simulink model "Batman_symbol"  (R2022a)
settings: Solver=VariableStepAuto  StartTime=0.0  StopTime=8  MaxStep=0.0001  RelTol=1e-3
libraries: simulink x8
settings Model: Creator=Gamer  LastModifiedBy=Gamer
settings SolverCC: ZeroCrossAlgorithm=Adaptive
settings DebuggingCC: IgnoredZcDiagnostic=none

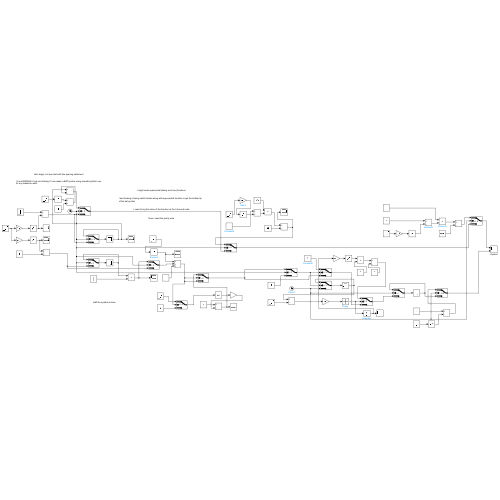
[thumbnail: Simulink's stored preview of the top-level diagram]
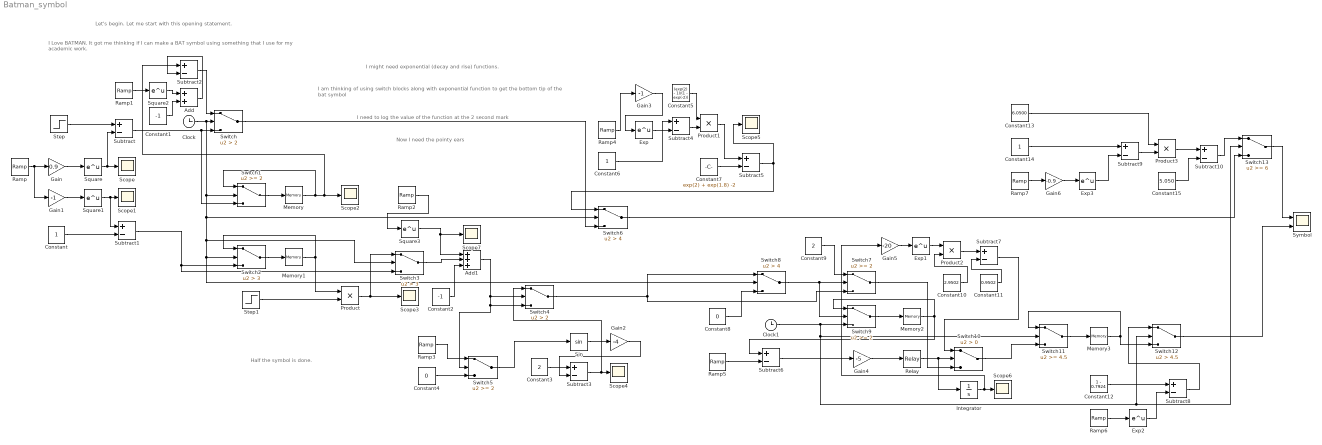
== system Batman_symbol ==
  note: Half the symbol is done.
  note: Now I need the pointy ears
  note: I need to log the value of the function at the 2 second mark
  note: I am thinking of using switch blocks along with exponential function to get the bottom tip of the bat symbol
  note: I might need exponential (decay and rise) functions.
  note: I Love BATMAN. It got me thinking if I can make a BAT symbol using something that I use for my academic work.
  note: Let's begin. Let me start with this opening statement.
  Add : Sum
  Add1 : Sum  Inputs=+++
  Clock : Clock
  Clock1 : Clock
  Constant : Constant
  Constant1 : Constant  Value=-1
  Constant10 : Constant  Value=2.9502
  Constant11 : Constant  Value=0.9502
  Constant12 : Constant  Value=1 - 0.7924
  Constant13 : Constant  Value=6.0500
  Constant14 : Constant
  Constant15 : Constant  Value=5.050
  Constant2 : Constant  Value=-1
  Constant3 : Constant  Value=2
  Constant4 : Constant  Value=0
  Constant5 : Constant  Value=(exp(2) - 1)/(1 - exp(-2))
  Constant6 : Constant
  Constant7 : Constant  Value=exp(2) + exp(1.8) -2
  Constant8 : Constant  Value=0
  Constant9 : Constant  Value=2
  Exp{,1..3} (4 alike) : Math
  Gain : Gain  Gain=0.9
  Gain1 : Gain  Gain=-1
  Gain2 : Gain  Gain=-4
  Gain3 : Gain  Gain=-1
  Gain4 : Gain  Gain=-5
  Gain5 : Gain  Gain=-20
  Gain6 : Gain  Gain=-0.9
  Integrator : Integrator
  Memory{,1..3} (4 alike) : Memory
  Product{,1..3} (4 alike) : Product
  Ramp : simulink/Sources/Ramp  slope=1  start=0  InitialOutput=0
  Ramp1 : simulink/Sources/Ramp  slope=1  start=2  InitialOutput=0
  Ramp2 : simulink/Sources/Ramp  slope=10  start=3.5  InitialOutput=0
  Ramp3 : simulink/Sources/Ramp  slope=4.33  start=0  InitialOutput=0
  Ramp4 : simulink/Sources/Ramp  slope=1  start=4  InitialOutput=0
  Ramp5 : simulink/Sources/Ramp  slope=1  start=0  InitialOutput=0
  Ramp6 : simulink/Sources/Ramp  slope=-0.449  start=4.5  InitialOutput=0
  Ramp7 : simulink/Sources/Ramp  slope=1  start=6  InitialOutput=0
  Relay : Relay  OnSwitchValue=0.001  OffSwitchValue=0
  Scope{,1..7} (8 alike) : Scope
  Sin : Trigonometry
  Square{,1..3} (4 alike) : Math
  Step : Step  Time=0  SampleTime=0
  Step1 : Step  Time=3  SampleTime=0
  Subtract{,1..10} (11 alike) : Sum  Inputs=+-
  Switch : Switch  Criteria=u2 > Threshold  Threshold=2  SaturateOnIntegerOverflow=off  InputSameDT=off
  Switch{1,5,7,9} (4 alike) : Switch  Threshold=2  SaturateOnIntegerOverflow=off  InputSameDT=off
  Switch10 : Switch  Criteria=u2 > Threshold  SaturateOnIntegerOverflow=off  InputSameDT=off
  Switch11 : Switch  Threshold=4.5  SaturateOnIntegerOverflow=off  InputSameDT=off
  Switch12 : Switch  Criteria=u2 > Threshold  Threshold=4.5  SaturateOnIntegerOverflow=off  InputSameDT=off
  Switch13 : Switch  Threshold=6  SaturateOnIntegerOverflow=off  InputSameDT=off
  Switch2 : Switch  Criteria=u2 > Threshold  Threshold=3  SaturateOnIntegerOverflow=off  InputSameDT=off
  Switch3 : Switch  Criteria=u2 > Threshold  Threshold=3  SaturateOnIntegerOverflow=off  InputSameDT=off
  Switch4 : Switch  Criteria=u2 > Threshold  Threshold=2  SaturateOnIntegerOverflow=off  InputSameDT=off
  Switch6 : Switch  Criteria=u2 > Threshold  Threshold=4  SaturateOnIntegerOverflow=off  InputSameDT=off
  Switch8 : Switch  Criteria=u2 > Threshold  Threshold=4  SaturateOnIntegerOverflow=off  InputSameDT=off
  Symbol : Scope  NumInputPorts=2
  wires:
  Step/1 -> Subtract/1
  Ramp/1 -> Gain1/1, Gain/1
  Square/1 -> Scope/1, Subtract/2
  Subtract/1 -> Switch1/3, Switch/3
  Gain/1 -> Square/1
  Gain1/1 -> Square1/1
  Square1/1 -> Subtract1/1, Scope1/1
  Constant/1 -> Subtract1/2
  Subtract1/1 -> Switch3/3, Switch2/3
  Clock/1 -> Switch8/2, Switch2/2, Switch3/2, Switch6/2, Switch1/2, Switch/2
  Ramp1/1 -> Square2/1
  Square2/1 -> Add/1
  Subtract2/1 -> Switch/1
  Switch1/1 -> Memory/1
  Memory/1 -> Subtract2/1, Scope2/1, Switch1/1
  Constant1/1 -> Add/2
  Add/1 -> Subtract2/2
  Switch2/1 -> Memory1/1
  Memory1/1 -> Switch2/1, Product/1
  Step1/1 -> Product/2
  Product/1 -> Switch3/1, Scope3/1
  Switch3/1 -> Add1/2
  Ramp2/1 -> Square3/1
  Square3/1 -> Scope7/1, Add1/1
  Add1/1 -> Switch5/2, Switch4/3, Switch4/2
  Constant2/1 -> Add1/3
  Switch4/1 -> Switch8/1, Switch7/3
  Switch5/1 -> Sin/1
  Constant3/1 -> Subtract3/1
  Subtract3/1 -> Switch4/1, Scope4/1
  Sin/1 -> Gain2/1
  Gain2/1 -> Subtract3/2
  Constant4/1 -> Switch5/3
  Ramp3/1 -> Switch5/1
  Switch/1 -> Switch6/3
  Ramp4/1 -> Gain3/1
  Gain3/1 -> Exp/1
  Exp/1 -> Subtract4/2
  Constant6/1 -> Subtract4/1
  Subtract4/1 -> Product1/2
  Constant5/1 -> Product1/1
  Product1/1 -> Subtract5/1
  Constant7/1 -> Subtract5/2
  Subtract5/1 -> Scope5/1, Switch6/1
  Switch6/1 -> Switch13/3
  Constant8/1 -> Switch8/3
  Switch8/1 -> Switch9/2, Switch7/2
  Constant9/1 -> Switch7/1
  Switch7/1 -> Switch10/3
  Clock1/1 -> Switch13/2, Switch12/2, Switch11/2, Switch9/3
  Switch9/1 -> Memory2/1
  Memory2/1 -> Subtract6/1, Switch9/1
  Ramp5/1 -> Subtract6/2
  Subtract6/1 -> Gain4/1
  Gain4/1 -> Relay/1
  Relay/1 -> Integrator/1, Switch10/2
  Switch10/1 -> Switch11/3
  Exp1/1 -> Product2/1
  Integrator/1 -> Gain5/1, Scope6/1
  Gain5/1 -> Exp1/1
  Product2/1 -> Subtract7/1
  Constant10/1 -> Product2/2
  Constant11/1 -> Subtract7/2
  Subtract7/1 -> Switch10/1
  Switch11/1 -> Memory3/1
  Memory3/1 -> Switch11/1, Switch12/3
  Ramp6/1 -> Exp2/1
  Constant12/1 -> Subtract8/1
  Exp2/1 -> Subtract8/2
  Subtract8/1 -> Switch12/1
  Switch12/1 -> Symbol/2
  Ramp7/1 -> Gain6/1
  Gain6/1 -> Exp3/1
  Constant14/1 -> Subtract9/1
  Exp3/1 -> Subtract9/2
  Subtract9/1 -> Product3/2
  Constant13/1 -> Product3/1
  Product3/1 -> Subtract10/1
  Constant15/1 -> Subtract10/2
  Subtract10/1 -> Switch13/1
  Switch13/1 -> Symbol/1
